simulink model "third"  (R2023b)
settings: Solver=FixedStepAuto  StartTime=0.0  StopTime=20  FixedStep=0.001  RelTol=1e-3
undefined symbols (not defined in the file): A1, A2, B1, B2, C1, C2, D1, D2, K1, K2, L1, L2, w0, w1, x0, x1
settings Model: Creator=evdokiiagalkina  LastModifiedBy=evdokiiagalkina

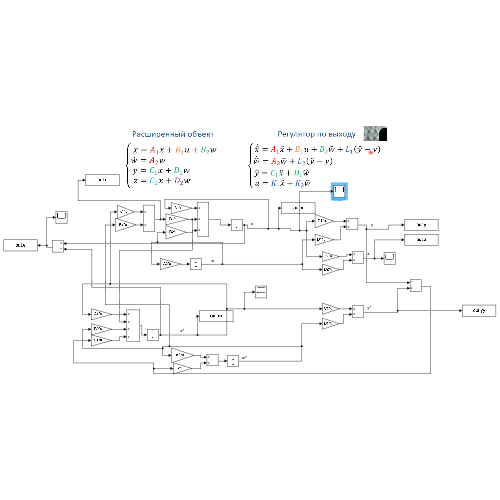
[thumbnail: Simulink's stored preview of the top-level diagram]
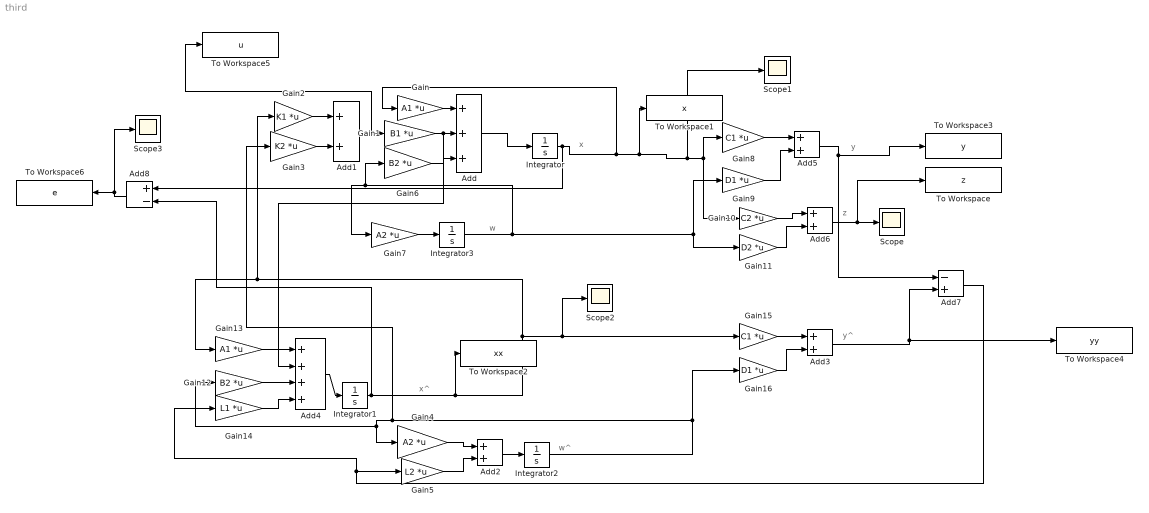
== system third ==
  note: z
  note: y
  note: x^
  note: w^
  note: x
  note: w
  note: y^
  Add : Sum  Inputs=+++
  Add{1..3,5..6} (5 alike) : Sum
  Add4 : Sum  Inputs=++++
  Add7 : Sum  Inputs=-+
  Add8 : Sum  Inputs=+-
  Gain : Gain  Gain=A1  Multiplication=Matrix(K*u)
  Gain1 : Gain  Gain=B1  Multiplication=Matrix(K*u)
  Gain10 : Gain  Gain=C2  Multiplication=Matrix(K*u)
  Gain11 : Gain  Gain=D2  Multiplication=Matrix(K*u)
  Gain12 : Gain  Gain=B2  Multiplication=Matrix(K*u)
  Gain13 : Gain  Gain=A1  Multiplication=Matrix(K*u)
  Gain14 : Gain  Gain=L1  Multiplication=Matrix(K*u)
  Gain15 : Gain  Gain=C1  Multiplication=Matrix(K*u)
  Gain16 : Gain  Gain=D1  Multiplication=Matrix(K*u)
  Gain2 : Gain  Gain=K1  Multiplication=Matrix(K*u)
  Gain3 : Gain  Gain=K2  Multiplication=Matrix(K*u)
  Gain4 : Gain  Gain=A2  Multiplication=Matrix(K*u)
  Gain5 : Gain  Gain=L2  Multiplication=Matrix(K*u)
  Gain6 : Gain  Gain=B2  Multiplication=Matrix(K*u)
  Gain7 : Gain  Gain=A2  Multiplication=Matrix(K*u)
  Gain8 : Gain  Gain=C1  Multiplication=Matrix(K*u)
  Gain9 : Gain  Gain=D1  Multiplication=Matrix(K*u)
  Integrator : Integrator  InitialCondition=x0
  Integrator1 : Integrator  InitialCondition=x1
  Integrator2 : Integrator  InitialCondition=w1
  Integrator3 : Integrator  InitialCondition=w0
  Scope{,1..3} (4 alike) : Scope
  To Workspace : ToWorkspace  VariableName=z  SaveFormat=Timeseries  SampleTime=-1
  To Workspace1 : ToWorkspace  VariableName=x  SaveFormat=Timeseries  SampleTime=-1
  To Workspace2 : ToWorkspace  VariableName=xx  SaveFormat=Timeseries  SampleTime=-1
  To Workspace3 : ToWorkspace  VariableName=y  SaveFormat=Timeseries  SampleTime=-1
  To Workspace4 : ToWorkspace  VariableName=yy  SaveFormat=Timeseries  SampleTime=-1
  To Workspace5 : ToWorkspace  VariableName=u  SaveFormat=Timeseries  SampleTime=-1
  To Workspace6 : ToWorkspace  VariableName=e  SaveFormat=Timeseries  SampleTime=-1
  wires:
  Add/1 -> Integrator/1
  Gain/1 -> Add/1
  Integrator/1 -> Add8/1, To Workspace1/1, Scope1/1, Gain8/1, Gain10/1, Gain/1
  Gain1/1 -> Add/2, Add4/2
  Gain2/1 -> Add1/1
  Gain3/1 -> Add1/2
  Add1/1 -> To Workspace5/1, Gain1/1
  Integrator1/1 -> Add8/2, To Workspace2/1, Scope2/1, Gain15/1, Gain13/1, Gain2/1
  Add2/1 -> Integrator2/1
  Gain4/1 -> Add2/1
  Integrator2/1 -> Gain16/1, Gain4/1, Gain12/1, Gain3/1
  Gain5/1 -> Add2/2
  Add3/1 -> Add7/2, To Workspace4/1
  Add4/1 -> Integrator1/1
  Gain6/1 -> Add/3
  Gain7/1 -> Integrator3/1
  Integrator3/1 -> Gain9/1, Gain11/1, Gain6/1, Gain7/1
  Gain8/1 -> Add5/1
  Gain9/1 -> Add5/2
  Add5/1 -> To Workspace3/1, Add7/1
  Gain10/1 -> Add6/1
  Add6/1 -> To Workspace/1, Scope/1
  Gain11/1 -> Add6/2
  Gain12/1 -> Add4/3
  Gain13/1 -> Add4/1
  Gain14/1 -> Add4/4
  Gain15/1 -> Add3/1
  Gain16/1 -> Add3/2
  Add7/1 -> Gain14/1, Gain5/1
  Add8/1 -> Scope3/1, To Workspace6/1
